simulink library "bcm"  (R2021b)
settings: Solver=VariableStepAuto  StartTime=0.0  StopTime=10.0  RelTol=1e-3
undefined symbols (not defined in the file or in its folder): ENUM_ANTITHEFT_ALARM, ENUM_ANTITHEFT_ARM, ENUM_ANTITHEFT_DISARM, ENUM_ANTITHEFT_WAIT, ENUM_GEARPOSNTOCAN_P, ENUM_PDKEYRAWLULOCK_INUNLOCK, ENUM_PDKEYRAWPS_INPS, ENUM_POWERSTA_ON, ENUM_POWERSTA_READY, ENUM_POWERSTA_STANDBY, FALSE, KBCM_ALMBrightnessDark_enum, KBCM_AmbBlue_enum, KBCM_AmbBreathT_ms, KBCM_AmbGreen_enum, KBCM_AmbRed_enum, KBCM_Antitheft_enum_ovrdflg, KBCM_Antitheft_enum_ovrdval, KBCM_APMDoorCtrlSta_flg_ovrdflg, KBCM_APMDoorCtrlSta_flg_ovrdval, KBCM_DelayTSW_flg, KBCM_DiagFLTC_mA, KBCM_DiagFMHT_s, KBCM_DiagFRTC_mA, KBCM_DiagRLTC_mA, KBCM_DiagRRTC_mA, KBCM_DrAPMRetryTimes_cnt, KBCM_DrOpenWdwOT_s, KBCM_DrOpenWdwReady_s, KBCM_ESSOffT_ms, KBCM_ESSOnT_ms, KBCM_IVIRstHoldT_ms, KBCM_IVIRstTriggerT_ms, KBCM_ONDelayT_ms, KBCM_ReDetectT_K, KBCM_RmLampKeep_min, KBCM_RmLpKeyInT_s, KBCM_RmLpKeyMissT_s, KBCM_SlpDebounceTime_s, KBCM_SPTGDetectT_sec, KBCM_SPTGLeave_flg, KBCM_SPTGLeftBound_cm, KBCM_SPTGLeftBoundOut_cm, KBCM_SPTGLowerBound_cm, KBCM_SPTGLowerBoundOut_cm, KBCM_SPTGRightBound_cm, KBCM_SPTGRightBoundOut_cm, KBCM_SPTGTOut_K, KBCM_SPTGUpperBound_cm, KBCM_SPTGUpperBoundOut_cm, KBCM_SPTGWaitDKC_sec, KBCM_TrunSWKeepTime3_s, KBCM_TrunSWKeepTime5_s, KBCM_TrunSWKeepTime7_s, KBCM_USSDis_cm, KBCM_USSFilterT_K, KBCM_WaitAPMPwr_K, KBCM_WdwManualDetT_s, MIN2SEC, TRUE ... (+1)
libraries: simulink x151, hcu_lib x5
(part 5 of 8)

== system bcm/BCM/BCM/PTG/KeyDetected ==
  VBCM_PASDRMR_cm : Inport
  VBCM_PASDRML_cm : Inport  Port=2
  AND{,1,3..4} (4 alike) : Logic  AllPortsSameDT=off  OutDataTypeStr=boolean
  AND2 : Logic  Inputs=3  AllPortsSameDT=off  OutDataTypeStr=boolean
  AND5 : Logic  Inputs=3  AllPortsSameDT=off  OutDataTypeStr=boolean
  Add : Sum
  Add1 : Sum  Inputs=-++
  Add2 : Sum  Inputs=--
  CheckSignalAvailable : Subsystem
  Compare To Constant2 : simulink/Logic and Bit Operations/Compare To Constant  relop=<=  const=KBCM_SPTGUpperBound_cm  OutDataTypeStr=boolean
  Compare To Constant3 : simulink/Logic and Bit Operations/Compare To Constant  relop=>=  const=KBCM_SPTGLowerBound_cm  OutDataTypeStr=boolean
  Constant : Constant  Value=KBCM_SPTGRightBound_cm
  Constant1 : Constant  Value=KBCM_USSFilterT_K
  Constant10 : Constant  Value=KBCM_USSDis_cm
  Constant11 : Constant  Value=KBCM_SPTGUpperBoundOut_cm
  Constant12 : Constant  Value=KBCM_SPTGLowerBoundOut_cm
  Constant13 : Constant  Value=KBCM_SPTGRightBoundOut_cm
  Constant14 : Constant  Value=KBCM_USSFilterT_K
  Constant15 : Constant  Value=-1  OutDataTypeStr=single
  Constant16 : Constant  Value=0  OutDataTypeStr=single
  Constant17 : Constant  Value=KBCM_SPTGUpperBound_cm
  Constant18 : Constant  Value=KBCM_SPTGLowerBound_cm
  Constant2 : Constant  Value=KBCM_SPTGLeftBound_cm
  Constant3 : Constant  Value=-1  OutDataTypeStr=single
  Constant4 : Constant  Value=KBCM_USSDis_cm
  Constant5 : Constant  Value=0  OutDataTypeStr=single
  Constant6 : Constant  Value=KBCM_SPTGLeftBoundOut_cm
  Constant7 : Constant  Value=KBCM_USSDis_cm
  Constant8 : Constant  Value=KBCM_SPTGLeftBound_cm
  Constant9 : Constant  Value=KBCM_SPTGLeftBound_cm
  Data Type Conversion : DataTypeConversion  OutDataTypeStr=single
  Data Type Conversion1 : DataTypeConversion  OutDataTypeStr=single
  Data Type Conversion2 : DataTypeConversion  OutDataTypeStr=boolean
  Data Type Conversion3 : DataTypeConversion  OutDataTypeStr=boolean
  Detect Decrease : simulink/Logic and Bit Operations/Detect Decrease  vinit=0.0  OutDataTypeStr=boolean
  Detect Decrease1 : simulink/Logic and Bit Operations/Detect Decrease  vinit=0.0  OutDataTypeStr=boolean
  Equal : RelationalOperator  OutDataTypeStr=boolean  RndMeth=Simplest
  Gain : Gain  Gain=-1
  GreaterThan : RelationalOperator  Operator=<=  OutDataTypeStr=boolean  RndMeth=Simplest
  GreaterThan1 : RelationalOperator  Operator=<=  OutDataTypeStr=boolean  RndMeth=Simplest
  GreaterThan2 : RelationalOperator  OutDataTypeStr=boolean  RndMeth=Simplest
  Less Than : RelationalOperator  Operator=<=  OutDataTypeStr=boolean  RndMeth=Simplest
  Less Than1 : RelationalOperator  OutDataTypeStr=boolean  RndMeth=Simplest
  Product : Product
  Sum1 : Sum
  Sum2 : Sum  Inputs=|++
  Sum3 : Sum  Inputs=|+-
  Sum4 : Sum
  Switch{1..6} (6 alike) : Switch  Criteria=u2 > Threshold
  Target_h : Subsystem
  Unit Delay{1..6} (6 alike) : UnitDelay  SampleTime=-1  HasFrameUpgradeWarning=on
  cosRML : Subsystem
  KeyDetected : Outport
  KeyDetectedOut : Outport  Port=2
  wires:
  Constant4/1 -> CheckSignalAvailable/3(KBCM_USSDis_cm_IN)
  CheckSignalAvailable/1(VBCM_PASDRML_cm) -> cosRML/1(VBCM_PASDRML_cm), Target_h/1(VBCM_PASDRML_cm), Product/2
  CheckSignalAvailable/2(VBCM_PASDRMR_cm) -> Target_h/2(VBCM_PASDRMR_cm), cosRML/2(VBCM_PASDRMR_cm)
  CheckSignalAvailable/3(KBCM_USSDis_cm) -> Target_h/3(KBCM_USSDis_cm), cosRML/3(KBCM_USSDis_cm)
  Target_h/1(Target_h) -> Less Than1/1, Less Than/1, Compare To Constant3/1, Compare To Constant2/1
  Compare To Constant2/1 -> AND1/1
  Compare To Constant3/1 -> AND1/2
  AND1/1 -> AND2/2
  AND/1 -> AND2/1
  cosRML/1(cosRML) -> Product/1
  CheckSignalAvailable/4(CheckResult) -> [CheckResult]
  [CheckResult] -> AND2/3
  Detect Decrease/1 -> Switch2/2
  Switch2/1 -> Data Type Conversion/1
  Constant1/1 -> Switch2/1
  Sum1/1 -> Switch2/3
  Unit Delay2/1 -> Switch3/2, Sum1/2, Switch4/2
  Constant3/1 -> Switch3/1
  Constant5/1 -> Switch3/3
  Switch3/1 -> Sum1/1
  Switch4/1 -> Data Type Conversion2/1, KeyDetected/1
  Unit Delay4/1 -> Switch4/1
  VBCM_PASDRML_cm/1 -> CheckSignalAvailable/1(VBCM_PASDRML_cm_IN)
  VBCM_PASDRMR_cm/1 -> CheckSignalAvailable/2(VBCM_PASDRMR_cm_IN)
  AND2/1 -> Unit Delay6/1, Detect Decrease/1
  GreaterThan1/1 -> AND4/1
  Add1/1 -> GreaterThan1/2
  [Target_x] -> GreaterThan2/1, GreaterThan1/1
  Product/1 -> [Target_x]
  [Target_x] -> GreaterThan/1, Equal/1
  Constant17/1 -> Sum2/1
  Constant11/1 -> Sum2/2
  Constant12/1 -> Sum3/2
  Constant18/1 -> Sum3/1
  [CheckResult] -> AND5/3
  AND3/1 -> AND5/1
  AND4/1 -> AND5/2
  AND5/1 -> Unit Delay1/1, Detect Decrease1/1
  Unit Delay5/1 -> Switch6/1
  Switch6/1 -> KeyDetectedOut/1, Data Type Conversion3/1
  Switch5/1 -> Sum4/1
  Constant16/1 -> Switch5/3
  Constant15/1 -> Switch5/1
  Unit Delay3/1 -> Switch6/2, Sum4/2, Switch5/2
  Sum4/1 -> Switch1/3
  Constant14/1 -> Switch1/1
  Switch1/1 -> Data Type Conversion1/1
  Detect Decrease1/1 -> Switch1/2
  Sum2/1 -> Less Than/2
  Less Than/1 -> AND3/1
  Sum3/1 -> Less Than1/2
  Less Than1/1 -> AND3/2
  Constant10/1 -> Add1/2
  Constant9/1 -> Add1/1
  Constant13/1 -> Add1/3
  Constant7/1 -> Add/2
  Equal/1 -> AND/1
  GreaterThan/1 -> AND/2
  Constant/1 -> Add/1
  Add/1 -> GreaterThan/2
  GreaterThan2/1 -> AND4/2
  Constant2/1 -> Add2/1
  Constant6/1 -> Add2/2
  Add2/1 -> GreaterThan2/2
  Unit Delay1/1 -> Switch6/3
  Unit Delay6/1 -> Switch4/3
  Constant8/1 -> Gain/1
  Gain/1 -> Equal/2
  Data Type Conversion/1 -> Unit Delay2/1
  Data Type Conversion1/1 -> Unit Delay3/1
  Data Type Conversion2/1 -> Unit Delay4/1
  Data Type Conversion3/1 -> Unit Delay5/1

== system bcm/BCM/BCM/PTG/Subsystem1 ==
  VAPM_PASDRMR_cm : Inport
  Add4 : Sum
  Compare To Constant1 : simulink/Logic and Bit Operations/Compare To Constant  relop=~=  const=0  OutDataTypeStr=boolean
  Compare To Constant6 : simulink/Logic and Bit Operations/Compare To Constant  relop===  const=0  OutDataTypeStr=boolean
  Compare To Constant8 : simulink/Logic and Bit Operations/Compare To Constant  relop===  const=255  OutDataTypeStr=boolean
  Constant1 : Constant  Value=0  OutDataTypeStr=uint8
  Constant12 : Constant  OutDataTypeStr=uint8
  Constant13 : Constant  Value=0  OutDataTypeStr=uint8
  Constant2 : Constant  OutDataTypeStr=uint8
  Constant3 : Constant  Value=KBCM_SPTGTOut_K
  Constant4 : Constant  Value=255  OutDataTypeStr=uint8
  Constant5 : Constant  Value=KBCM_SPTGTOut_K
  Detect Change : simulink/Logic and Bit Operations/Detect Change  vinit=0  OutDataTypeStr=boolean
  Equal : RelationalOperator  OutDataTypeStr=boolean  RndMeth=Simplest
  Equal1 : RelationalOperator  Operator===  OutDataTypeStr=boolean  RndMeth=Simplest
  Equal2 : RelationalOperator  Operator=~=  OutDataTypeStr=boolean  RndMeth=Simplest
  Logical Operator : Logic  Inputs=3  AllPortsSameDT=off  OutDataTypeStr=boolean
  Logical Operator2 : Logic  Operator=OR  AllPortsSameDT=off  OutDataTypeStr=boolean
  Switch{2..3,8..9} (4 alike) : Switch  Criteria=u2 > Threshold
  Unit Delay2 : UnitDelay  SampleTime=-1  HasFrameUpgradeWarning=on
  Unit Delay6 : UnitDelay  SampleTime=-1  HasFrameUpgradeWarning=on
  PASDRMR : Outport
  wires:
  Equal1/1 -> Logical Operator2/2
  Switch9/1 -> Add4/1
  Constant5/1 -> Equal1/1, Equal2/2
  Unit Delay6/1 -> Equal/1, Add4/2
  Compare To Constant8/1 -> Switch8/2
  Equal2/1 -> Logical Operator2/1
  Constant4/1 -> Switch3/3
  Switch2/1 -> Switch3/1, Unit Delay2/1
  Compare To Constant1/1 -> Logical Operator/2
  Logical Operator/1 -> Switch2/2
  Constant13/1 -> Switch9/1
  Add4/1 -> Switch8/1
  Unit Delay2/1 -> Switch2/3
  Constant12/1 -> Switch9/3
  Equal/1 -> Switch9/2
  Constant3/1 -> Equal/2
  Detect Change/1 -> Logical Operator/1
  Compare To Constant6/1 -> Logical Operator/3
  Constant1/1 -> Switch8/3
  Switch3/1 -> PASDRMR/1
  VAPM_PASDRMR_cm/1 -> Switch2/1, Detect Change/1, Compare To Constant1/1, Compare To Constant8/1
  Logical Operator2/1 -> Switch3/2
  Constant2/1 -> Equal1/2
  Switch8/1 -> Unit Delay6/1, Compare To Constant6/1, Equal2/1

== system bcm/BCM/BCM/PTG/Subsystem3 ==
  VAPM_PASDRML_cm : Inport
  Add4 : Sum
  Compare To Constant1 : simulink/Logic and Bit Operations/Compare To Constant  relop=~=  const=0  OutDataTypeStr=boolean
  Compare To Constant6 : simulink/Logic and Bit Operations/Compare To Constant  relop===  const=0  OutDataTypeStr=boolean
  Compare To Constant8 : simulink/Logic and Bit Operations/Compare To Constant  relop===  const=255  OutDataTypeStr=boolean
  Constant1 : Constant  Value=0  OutDataTypeStr=uint8
  Constant12 : Constant  OutDataTypeStr=uint8
  Constant13 : Constant  Value=0  OutDataTypeStr=uint8
  Constant2 : Constant  Value=0  OutDataTypeStr=uint8
  Constant3 : Constant  Value=KBCM_SPTGTOut_K
  Constant4 : Constant  Value=255  OutDataTypeStr=uint8
  Constant5 : Constant  Value=KBCM_SPTGTOut_K
  Detect Change : simulink/Logic and Bit Operations/Detect Change  vinit=0  OutDataTypeStr=boolean
  Equal : RelationalOperator  OutDataTypeStr=boolean  RndMeth=Simplest
  Equal1 : RelationalOperator  Operator===  OutDataTypeStr=boolean  RndMeth=Simplest
  Equal2 : RelationalOperator  Operator=~=  OutDataTypeStr=boolean  RndMeth=Simplest
  Logical Operator : Logic  Inputs=3  AllPortsSameDT=off  OutDataTypeStr=boolean
  Logical Operator2 : Logic  Operator=OR  AllPortsSameDT=off  OutDataTypeStr=boolean
  Switch{2..3,8..9} (4 alike) : Switch  Criteria=u2 > Threshold
  Unit Delay2 : UnitDelay  SampleTime=-1  HasFrameUpgradeWarning=on
  Unit Delay6 : UnitDelay  SampleTime=-1  HasFrameUpgradeWarning=on
  PASDRML : Outport
  wires:
  Constant2/1 -> Equal1/2
  Logical Operator2/1 -> Switch3/2
  VAPM_PASDRML_cm/1 -> Compare To Constant8/1, Compare To Constant1/1, Detect Change/1, Switch2/1
  Switch3/1 -> PASDRML/1
  Constant1/1 -> Switch8/3
  Compare To Constant6/1 -> Logical Operator/3
  Detect Change/1 -> Logical Operator/1
  Constant3/1 -> Equal/2
  Equal/1 -> Switch9/2
  Constant12/1 -> Switch9/3
  Unit Delay2/1 -> Switch2/3
  Add4/1 -> Switch8/1
  Constant13/1 -> Switch9/1
  Switch8/1 -> Equal2/1, Compare To Constant6/1, Unit Delay6/1
  Logical Operator/1 -> Switch2/2
  Compare To Constant1/1 -> Logical Operator/2
  Switch2/1 -> Unit Delay2/1, Switch3/1
  Constant4/1 -> Switch3/3
  Equal2/1 -> Logical Operator2/1
  Compare To Constant8/1 -> Switch8/2
  Unit Delay6/1 -> Add4/2, Equal/1
  Constant5/1 -> Equal2/2, Equal1/1
  Switch9/1 -> Add4/1
  Equal1/1 -> Logical Operator2/2

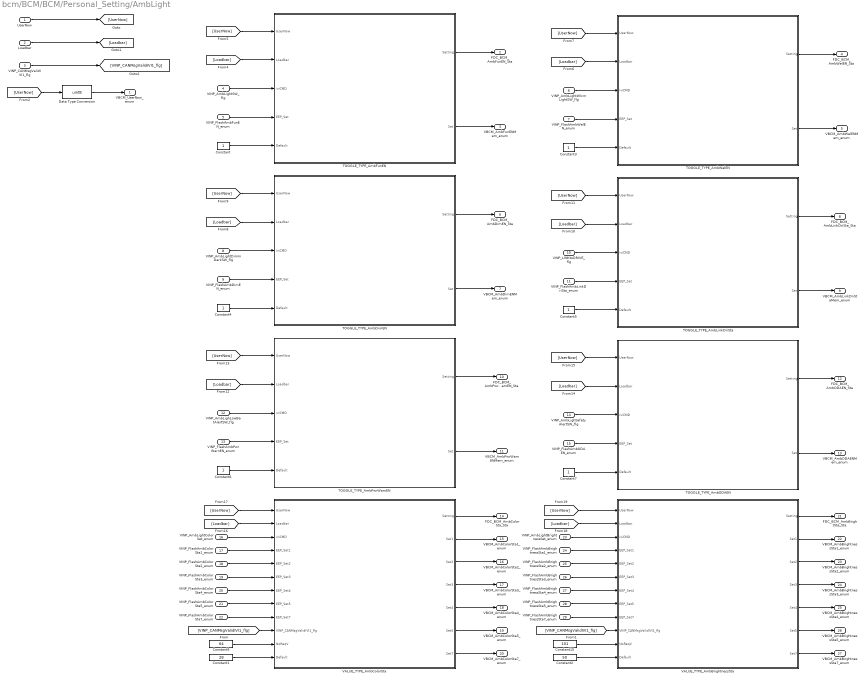
== system bcm/BCM/BCM/Personal_Setting/AmbLight ==
  UserNow : Inport
  Loadbar : Inport  Port=2
  VINP_CANMsgValidIVI1_flg : Inport  Port=3
  VINP_AmbLightSW_flg : Inport  Port=4
  VINP_FlashAmbFunEN_enum : Inport  Port=5
  VINP_AmbLightWlcmLightSW_flg : Inport  Port=6
  VINP_FlashAmbWelEN_enum : Inport  Port=7
  VINP_AmbLightDimInDarkSW_flg : Inport  Port=8
  VINP_FlashAmbDimEN_enum : Inport  Port=9
  VINP_LINKtoDRIVE_flg : Inport  Port=10
  VINP_FlashAmbLinkDriSta_enum : Inport  Port=11
  VINP_AmbLighLowBatAlertSW_flg : Inport  Port=12
  VINP_FlashAmbPwrWarnEN_enum : Inport  Port=13
  VINP_AmbLighSafetyAlertSW_flg : Inport  Port=14
  VINP_FlashAmbODAEN_enum : Inport  Port=15
  VINP_AmbLightColorSet_enum : Inport  Port=16
  VINP_FlashAmbColorSta1_enum : Inport  Port=17
  VINP_FlashAmbColorSta2_enum : Inport  Port=18
  VINP_FlashAmbColorSta3_enum : Inport  Port=19
  VINP_FlashAmbColorSta4_enum : Inport  Port=20
  VINP_FlashAmbColorSta5_enum : Inport  Port=21
  VINP_FlashAmbColorSta7_enum : Inport  Port=22
  VINP_AmbLightBrightnessSet_enum : Inport  Port=23
  VINP_FlashAmbBrightnessSta1_enum : Inport  Port=24
  VINP_FlashAmbBrightnessSta2_enum : Inport  Port=25
  VINP_FlashAmbBrightnessSta3_enum : Inport  Port=26
  VINP_FlashAmbBrightnessSta4_enum : Inport  Port=27
  VINP_FlashAmbBrightnessSta5_enum : Inport  Port=28
  VINP_FlashAmbBrightnessSta7_enum : Inport  Port=29
  Constant{,3..7} (6 alike) : Constant  OutDataTypeStr=boolean
  Constant1 : Constant  Value=28  OutDataTypeStr=uint8
  Constant10 : Constant  Value=101  OutDataTypeStr=uint8
  Constant2 : Constant  Value=50  OutDataTypeStr=uint8
  Constant9 : Constant  Value=64  OutDataTypeStr=uint8
  Data Type Conversion : DataTypeConversion  OutDataTypeStr=uint8
  TOGGLE_TYPE_AmbDimEN : Subsystem
  TOGGLE_TYPE_AmbFunEN : Subsystem
  TOGGLE_TYPE_AmbLinkDriSta : Subsystem
  TOGGLE_TYPE_AmbODAEN : Subsystem
  TOGGLE_TYPE_AmbPwrWarnEN : Subsystem
  TOGGLE_TYPE_AmbWelEN : Subsystem
  VALUE_TYPE_AmbBrightnessSta : Subsystem
  VALUE_TYPE_AmbColorSta : Subsystem
  VBCM_UserNow_enum : Outport
  FDC_BCM_AmbFunEN_Sta : Outport  Port=2
  VBCM_AmbFunENMem_enum : Outport  Port=3
  FDC_BCM_AmbWelEN_Sta : Outport  Port=4
  VBCM_AmbWelENMem_enum : Outport  Port=5
  FDC_BCM_AmbDimEN_Sta : Outport  Port=6
  VBCM_AmbDimENMem_enum : Outport  Port=7
  FDC_BCM_AmbLinkDriSta_Sta : Outport  Port=8
  VBCM_AmbLinkDriStaMem_enum : Outport  Port=9
  FDC_BCM_AmbPwrWarnEN_Sta : Outport  Port=10
  VBCM_AmbPwrWarnENMem_enum : Outport  Port=11
  FDC_BCM_AmbODAEN_Sta : Outport  Port=12
  VBCM_AmbODAENMem_enum : Outport  Port=13
  FDC_BCM_AmbColorSta_Sta : Outport  Port=14
  VBCM_AmbColorSta1_enum : Outport  Port=15
  VBCM_AmbColorSta2_enum : Outport  Port=16
  VBCM_AmbColorSta3_enum : Outport  Port=17
  VBCM_AmbColorSta4_enum : Outport  Port=18
  VBCM_AmbColorSta5_enum : Outport  Port=19
  VBCM_AmbColorSta7_enum : Outport  Port=20
  FDC_BCM_AmbBrightSta_Sta : Outport  Port=21  OutDataTypeStr=uint8
  VBCM_AmbBrightnessSta1_enum : Outport  Port=22  OutDataTypeStr=uint8
  VBCM_AmbBrightnessSta2_enum : Outport  Port=23
  VBCM_AmbBrightnessSta3_enum : Outport  Port=24
  VBCM_AmbBrightnessSta4_enum : Outport  Port=25
  VBCM_AmbBrightnessSta5_enum : Outport  Port=26
  VBCM_AmbBrightnessSta7_enum : Outport  Port=27
  wires:
  VALUE_TYPE_AmbBrightnessSta/3(Set2) -> VBCM_AmbBrightnessSta2_enum/1
  VALUE_TYPE_AmbBrightnessSta/2(Set1) -> VBCM_AmbBrightnessSta1_enum/1
  [UserNow] -> VALUE_TYPE_AmbBrightnessSta/1(UserNow)
  VALUE_TYPE_AmbBrightnessSta/1(Setting) -> FDC_BCM_AmbBrightSta_Sta/1
  TOGGLE_TYPE_AmbFunEN/1(Setting) -> FDC_BCM_AmbFunEN_Sta/1
  [Loadbar] -> VALUE_TYPE_AmbColorSta/2(Loadbar)
  VALUE_TYPE_AmbBrightnessSta/6(Set5) -> VBCM_AmbBrightnessSta5_enum/1
  TOGGLE_TYPE_AmbFunEN/2(Set) -> VBCM_AmbFunENMem_enum/1
  VALUE_TYPE_AmbBrightnessSta/7(Set7) -> VBCM_AmbBrightnessSta7_enum/1
  VALUE_TYPE_AmbBrightnessSta/4(Set3) -> VBCM_AmbBrightnessSta3_enum/1
  [UserNow] -> VALUE_TYPE_AmbColorSta/1(UserNow)
  VALUE_TYPE_AmbBrightnessSta/5(Set4) -> VBCM_AmbBrightnessSta4_enum/1
  [Loadbar] -> VALUE_TYPE_AmbBrightnessSta/2(Loadbar)
  UserNow/1 -> [UserNow]
  Loadbar/1 -> [Loadbar]
  VALUE_TYPE_AmbColorSta/1(Setting) -> FDC_BCM_AmbColorSta_Sta/1
  VALUE_TYPE_AmbColorSta/2(Set1) -> VBCM_AmbColorSta1_enum/1
  VALUE_TYPE_AmbColorSta/3(Set2) -> VBCM_AmbColorSta2_enum/1
  VALUE_TYPE_AmbColorSta/4(Set3) -> VBCM_AmbColorSta3_enum/1
  VALUE_TYPE_AmbColorSta/5(Set4) -> VBCM_AmbColorSta4_enum/1
  VALUE_TYPE_AmbColorSta/6(Set5) -> VBCM_AmbColorSta5_enum/1
  VALUE_TYPE_AmbColorSta/7(Set7) -> VBCM_AmbColorSta7_enum/1
  [UserNow] -> TOGGLE_TYPE_AmbFunEN/1(UserNow)
  [Loadbar] -> TOGGLE_TYPE_AmbFunEN/2(Loadbar)
  VINP_AmbLightSW_flg/1 -> TOGGLE_TYPE_AmbFunEN/3(iviCMD)
  VINP_FlashAmbFunEN_enum/1 -> TOGGLE_TYPE_AmbFunEN/4(EEP_Set)
  Constant/1 -> TOGGLE_TYPE_AmbFunEN/5(Default)
  Constant9/1 -> VALUE_TYPE_AmbColorSta/11(NoReqV)
  Constant1/1 -> VALUE_TYPE_AmbColorSta/12(Default)
  VINP_FlashAmbColorSta7_enum/1 -> VALUE_TYPE_AmbColorSta/9(EEP_Set7)
  VINP_FlashAmbColorSta5_enum/1 -> VALUE_TYPE_AmbColorSta/8(EEP_Set5)
  VINP_FlashAmbColorSta4_enum/1 -> VALUE_TYPE_AmbColorSta/7(EEP_Set4)
  VINP_FlashAmbColorSta3_enum/1 -> VALUE_TYPE_AmbColorSta/6(EEP_Set3)
  VINP_FlashAmbColorSta2_enum/1 -> VALUE_TYPE_AmbColorSta/5(EEP_Set2)
  VINP_FlashAmbColorSta1_enum/1 -> VALUE_TYPE_AmbColorSta/4(EEP_Set1)
  VINP_AmbLightColorSet_enum/1 -> VALUE_TYPE_AmbColorSta/3(iviCMD)
  Constant10/1 -> VALUE_TYPE_AmbBrightnessSta/11(NoReqV)
  Constant2/1 -> VALUE_TYPE_AmbBrightnessSta/12(Default)
  VINP_FlashAmbBrightnessSta7_enum/1 -> VALUE_TYPE_AmbBrightnessSta/9(EEP_Set7)
  VINP_FlashAmbBrightnessSta5_enum/1 -> VALUE_TYPE_AmbBrightnessSta/8(EEP_Set5)
  VINP_FlashAmbBrightnessSta4_enum/1 -> VALUE_TYPE_AmbBrightnessSta/7(EEP_Set4)
  VINP_FlashAmbBrightnessSta3_enum/1 -> VALUE_TYPE_AmbBrightnessSta/6(EEP_Set3)
  VINP_FlashAmbBrightnessSta2_enum/1 -> VALUE_TYPE_AmbBrightnessSta/5(EEP_Set2)
  VINP_FlashAmbBrightnessSta1_enum/1 -> VALUE_TYPE_AmbBrightnessSta/4(EEP_Set1)
  VINP_AmbLightBrightnessSet_enum/1 -> VALUE_TYPE_AmbBrightnessSta/3(iviCMD)
  [UserNow] -> TOGGLE_TYPE_AmbWelEN/1(UserNow)
  [Loadbar] -> TOGGLE_TYPE_AmbWelEN/2(Loadbar)
  Constant3/1 -> TOGGLE_TYPE_AmbWelEN/5(Default)
  VINP_AmbLightWlcmLightSW_flg/1 -> TOGGLE_TYPE_AmbWelEN/3(iviCMD)
  VINP_FlashAmbWelEN_enum/1 -> TOGGLE_TYPE_AmbWelEN/4(EEP_Set)
  TOGGLE_TYPE_AmbWelEN/1(Setting) -> FDC_BCM_AmbWelEN_Sta/1
  TOGGLE_TYPE_AmbWelEN/2(Set) -> VBCM_AmbWelENMem_enum/1
  [UserNow] -> TOGGLE_TYPE_AmbDimEN/1(UserNow)
  Constant4/1 -> TOGGLE_TYPE_AmbDimEN/5(Default)
  [Loadbar] -> TOGGLE_TYPE_AmbDimEN/2(Loadbar)
  VINP_AmbLightDimInDarkSW_flg/1 -> TOGGLE_TYPE_AmbDimEN/3(iviCMD)
  VINP_FlashAmbDimEN_enum/1 -> TOGGLE_TYPE_AmbDimEN/4(EEP_Set)
  TOGGLE_TYPE_AmbDimEN/1(Setting) -> FDC_BCM_AmbDimEN_Sta/1
  TOGGLE_TYPE_AmbDimEN/2(Set) -> VBCM_AmbDimENMem_enum/1
  [UserNow] -> TOGGLE_TYPE_AmbLinkDriSta/1(UserNow)
  Constant5/1 -> TOGGLE_TYPE_AmbLinkDriSta/5(Default)
  [Loadbar] -> TOGGLE_TYPE_AmbLinkDriSta/2(Loadbar)
  VINP_LINKtoDRIVE_flg/1 -> TOGGLE_TYPE_AmbLinkDriSta/3(iviCMD)
  VINP_FlashAmbLinkDriSta_enum/1 -> TOGGLE_TYPE_AmbLinkDriSta/4(EEP_Set)
  TOGGLE_TYPE_AmbLinkDriSta/1(Setting) -> FDC_BCM_AmbLinkDriSta_Sta/1
  TOGGLE_TYPE_AmbLinkDriSta/2(Set) -> VBCM_AmbLinkDriStaMem_enum/1
  Constant6/1 -> TOGGLE_TYPE_AmbPwrWarnEN/5(Default)
  [UserNow] -> TOGGLE_TYPE_AmbPwrWarnEN/1(UserNow)
  [Loadbar] -> TOGGLE_TYPE_AmbPwrWarnEN/2(Loadbar)
  VINP_AmbLighLowBatAlertSW_flg/1 -> TOGGLE_TYPE_AmbPwrWarnEN/3(iviCMD)
  VINP_FlashAmbPwrWarnEN_enum/1 -> TOGGLE_TYPE_AmbPwrWarnEN/4(EEP_Set)
  TOGGLE_TYPE_AmbPwrWarnEN/1(Setting) -> FDC_BCM_AmbPwrWarnEN_Sta/1
  TOGGLE_TYPE_AmbPwrWarnEN/2(Set) -> VBCM_AmbPwrWarnENMem_enum/1
  [UserNow] -> TOGGLE_TYPE_AmbODAEN/1(UserNow)
  [Loadbar] -> TOGGLE_TYPE_AmbODAEN/2(Loadbar)
  Constant7/1 -> TOGGLE_TYPE_AmbODAEN/5(Default)
  VINP_AmbLighSafetyAlertSW_flg/1 -> TOGGLE_TYPE_AmbODAEN/3(iviCMD)
  VINP_FlashAmbODAEN_enum/1 -> TOGGLE_TYPE_AmbODAEN/4(EEP_Set)
  TOGGLE_TYPE_AmbODAEN/1(Setting) -> FDC_BCM_AmbODAEN_Sta/1
  TOGGLE_TYPE_AmbODAEN/2(Set) -> VBCM_AmbODAENMem_enum/1
  VINP_CANMsgValidIVI1_flg/1 -> [VINP_CANMsgValidIVI1_flg]
  [VINP_CANMsgValidIVI1_flg] -> VALUE_TYPE_AmbColorSta/10(VINP_CANMsgValidIVI1_flg)
  [VINP_CANMsgValidIVI1_flg] -> VALUE_TYPE_AmbBrightnessSta/10(VINP_CANMsgValidIVI1_flg)
  [UserNow] -> Data Type Conversion/1
  Data Type Conversion/1 -> VBCM_UserNow_enum/1

== system bcm/BCM/BCM/Personal_Setting/System_Loadbar ==
  Add : Sum
  Compare To Constant : simulink/Logic and Bit Operations/Compare To Constant  relop=>  const=2  OutDataTypeStr=boolean
  Constant6 : Constant  Value=0  OutDataTypeStr=uint8
  Constant7 : Constant  OutDataTypeStr=uint8
  Switch7 : Switch  Criteria=u2 > Threshold
  Unit Delay : UnitDelay  SampleTime=-1  HasFrameUpgradeWarning=on
  Unit Delay6 : UnitDelay  SampleTime=-1  HasFrameUpgradeWarning=on
  Loadbar : Outport
  wires:
  Constant7/1 -> Switch7/3
  Unit Delay6/1 -> Add/1
  Switch7/1 -> Add/2
  Unit Delay/1 -> Switch7/2
  Compare To Constant/1 -> Unit Delay/1, Loadbar/1
  Add/1 -> Unit Delay6/1, Compare To Constant/1
  Constant6/1 -> Switch7/1

== system bcm/BCM/BCM/PTG/KeyDetected/CheckSignalAvailable ==
  VBCM_PASDRML_cm_IN : Inport
  VBCM_PASDRMR_cm_IN : Inport  Port=2
  KBCM_USSDis_cm_IN : Inport  Port=3
  AND : Logic  Inputs=3  AllPortsSameDT=off  OutDataTypeStr=boolean
  Constant : Constant  OutDataTypeStr=single
  Constant1 : Constant  OutDataTypeStr=single
  Constant2 : Constant  OutDataTypeStr=single
  Constant3 : Constant  Value=KBCM_SPTGLowerBound_cm
  Constant4 : Constant  Value=KBCM_SPTGLowerBoundOut_cm
  Constant5 : Constant  Value=KBCM_SPTGLowerBound_cm
  Constant6 : Constant  Value=KBCM_SPTGLowerBoundOut_cm
  Demux : Demux  Outputs=3
  Equal : RelationalOperator  OutDataTypeStr=boolean  RndMeth=Simplest
  Equal1 : RelationalOperator  OutDataTypeStr=boolean  RndMeth=Simplest
  GreaterThan : RelationalOperator  OutDataTypeStr=boolean  RndMeth=Simplest
  Max : MinMax  Function=max  Inputs=3
  Mux : Mux  Inputs=3
  Mux1 : Mux  Inputs=3
  Sum : Sum  Inputs=+-
  Sum1 : Sum  Inputs=+++
  Sum2 : Sum  Inputs=|+-
  Sum3 : Sum  Inputs=|+-
  Switch : Switch  Criteria=u2 > Threshold
  VBCM_PASDRML_cm : Outport
  VBCM_PASDRMR_cm : Outport  Port=2
  KBCM_USSDis_cm : Outport  Port=3
  CheckResult : Outport  Port=4
  wires:
  GreaterThan/1 -> AND/1
  VBCM_PASDRML_cm_IN/1 -> [VBCM_PASDRML_cm_IN]
  VBCM_PASDRMR_cm_IN/1 -> [VBCM_PASDRMR_cm_IN]
  KBCM_USSDis_cm_IN/1 -> [KBCM_USSDis_cm_IN]
  AND/1 -> Switch/2, CheckResult/1
  Mux/1 -> Switch/1
  [VBCM_PASDRML_cm_IN] -> Mux/1
  [VBCM_PASDRMR_cm_IN] -> Mux/2
  [KBCM_USSDis_cm_IN] -> Mux/3
  Mux1/1 -> Switch/3
  Constant/1 -> Mux1/1
  Constant1/1 -> Mux1/2
  Switch/1 -> Demux/1
  Demux/1 -> VBCM_PASDRML_cm/1
  Demux/2 -> VBCM_PASDRMR_cm/1
  Demux/3 -> KBCM_USSDis_cm/1
  Equal/1 -> AND/2
  [VBCM_PASDRML_cm_IN] -> Max/1, Sum1/1
  [VBCM_PASDRMR_cm_IN] -> Max/2, Sum1/2
  [KBCM_USSDis_cm_IN] -> Max/3, Sum1/3
  Sum1/1 -> Sum/1
  Max/1 -> Sum/2, GreaterThan/2
  Sum/1 -> GreaterThan/1
  Constant2/1 -> Mux1/3
  Equal1/1 -> AND/3
  [VBCM_PASDRMR_cm_IN] -> Equal/1
  Constant3/1 -> Sum2/1
  Constant4/1 -> Sum2/2
  Sum2/1 -> Equal/2
  Sum3/1 -> Equal1/2
  Constant6/1 -> Sum3/2
  Constant5/1 -> Sum3/1
  [VBCM_PASDRML_cm_IN] -> Equal1/1

== system bcm/BCM/BCM/PTG/KeyDetected/Target_h ==
  VBCM_PASDRML_cm : Inport
  VBCM_PASDRMR_cm : Inport  Port=2
  KBCM_USSDis_cm : Inport  Port=3
  Data Type Conversion : DataTypeConversion
  Divide : Product  Inputs=*/
  Gain : Gain  Gain=2
  Gain1 : Gain  Gain=0.5
  Product : Product  Inputs=4
  Sqrt1 : Sqrt  SaturateOnIntegerOverflow=on
  Sum : Sum  Inputs=+-
  Sum1 : Sum  Inputs=+++
  Sum2 : Sum  Inputs=+-
  Sum3 : Sum  Inputs=+-
  Terminator : Terminator
  Target_h : Outport
  wires:
  Divide/1 -> Data Type Conversion/1, Target_h/1
  VBCM_PASDRML_cm/1 -> Sum/2, Sum1/1
  VBCM_PASDRMR_cm/1 -> Sum2/2, Sum1/2
  KBCM_USSDis_cm/1 -> Divide/2, Sum3/2, Sum1/3
  Sum1/1 -> Gain1/1
  Sum/1 -> Product/2
  Sum2/1 -> Product/3
  Sum3/1 -> Product/4
  Product/1 -> Sqrt1/1
  Sqrt1/1 -> Gain/1
  Gain/1 -> Divide/1
  Gain1/1 -> Sum3/1, Sum2/1, Sum/1, Product/1
  Data Type Conversion/1 -> Terminator/1  "VBCM_Targeth_cm"

== system bcm/BCM/BCM/PTG/KeyDetected/cosRML ==
  VBCM_PASDRML_cm : Inport
  VBCM_PASDRMR_cm : Inport  Port=2
  KBCM_USSDis_cm : Inport  Port=3
  Divide : Product  Inputs=*/
  Gain : Gain  Gain=2
  Product : Product
  Square : Math  Operator=square  SaturateOnIntegerOverflow=on
  Square1 : Math  Operator=square  SaturateOnIntegerOverflow=on
  Square2 : Math  Operator=square  SaturateOnIntegerOverflow=on
  Sum : Sum  Inputs=+-+
  cosRML : Outport
  wires:
  VBCM_PASDRML_cm/1 -> Product/1, Square/1
  VBCM_PASDRMR_cm/1 -> Square1/1
  KBCM_USSDis_cm/1 -> Product/2, Square2/1
  Square/1 -> Sum/1
  Square1/1 -> Sum/2
  Square2/1 -> Sum/3
  Product/1 -> Gain/1
  Sum/1 -> Divide/1
  Divide/1 -> cosRML/1
  Gain/1 -> Divide/2

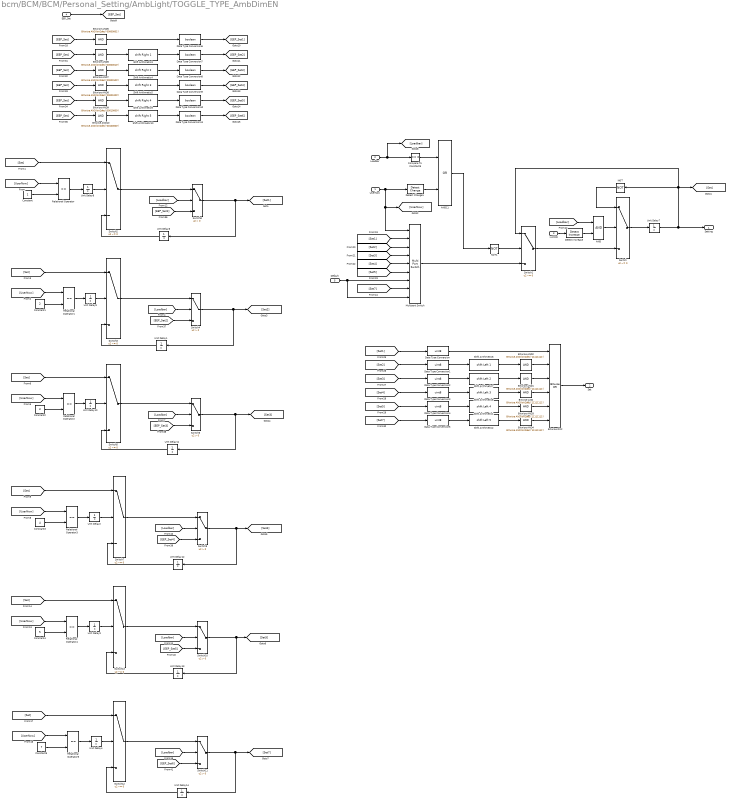
== system bcm/BCM/BCM/Personal_Setting/AmbLight/TOGGLE_TYPE_AmbDimEN ==
  UserNow : Inport
  Loadbar : Inport  Port=2
  iviCMD : Inport  Port=3
  EEP_Set : Inport  Port=4
  Default : Inport  Port=5
  AND : Logic  AllPortsSameDT=off  OutDataTypeStr=boolean
  AND11 : Logic  Operator=OR  AllPortsSameDT=off  OutDataTypeStr=boolean
  Bitwise AND{,1..4} (5 alike) : simulink/Logic and Bit Operations/Bitwise Operator  logicop=AND  UseBitMask=on  BitMask=bin2dec('11111111')  BitMaskRealWorld=Stored Integer
  Bitwise AND10 : simulink/Logic and Bit Operations/Bitwise Operator  logicop=AND  UseBitMask=on  BitMask=bin2dec('00100000')  BitMaskRealWorld=Stored Integer
  Bitwise AND5 : simulink/Logic and Bit Operations/Bitwise Operator  logicop=AND  UseBitMask=on  BitMask=bin2dec('00000001')  BitMaskRealWorld=Stored Integer
  Bitwise AND6 : simulink/Logic and Bit Operations/Bitwise Operator  logicop=AND  UseBitMask=on  BitMask=bin2dec('00000010')  BitMaskRealWorld=Stored Integer
  Bitwise AND7 : simulink/Logic and Bit Operations/Bitwise Operator  logicop=AND  UseBitMask=on  BitMask=bin2dec('00000100')  BitMaskRealWorld=Stored Integer
  Bitwise AND8 : simulink/Logic and Bit Operations/Bitwise Operator  logicop=AND  UseBitMask=on  BitMask=bin2dec('00001000')  BitMaskRealWorld=Stored Integer
  Bitwise AND9 : simulink/Logic and Bit Operations/Bitwise Operator  logicop=AND  UseBitMask=on  BitMask=bin2dec('00010000')  BitMaskRealWorld=Stored Integer
  Bitwise OR2 : simulink/Logic and Bit Operations/Bitwise Operator  logicop=OR  UseBitMask=off  NumInputPorts=6  BitMask=bin2dec('00000000000000000000')  BitMaskRealWorld=Stored Integer
  Compare To Constant5 : simulink/Logic and Bit Operations/Compare To Constant  relop===  const=0  OutDataTypeStr=boolean
  Constant : Constant  OutDataTypeStr=uint8
  Constant1 : Constant  Value=2  OutDataTypeStr=uint8
  Constant2 : Constant  Value=3  OutDataTypeStr=uint8
  Constant3 : Constant  Value=4  OutDataTypeStr=uint8
  Constant4 : Constant  Value=5  OutDataTypeStr=uint8
  Constant5 : Constant  Value=7  OutDataTypeStr=uint8
  Data Type Conversion{,1..5} (6 alike) : DataTypeConversion  OutDataTypeStr=uint8
  Data Type Conversion{6..11} (6 alike) : DataTypeConversion  OutDataTypeStr=boolean
  Detect Change1 : simulink/Logic and Bit Operations/Detect Change  vinit=0  OutDataTypeStr=boolean
  Detect Increase : simulink/Logic and Bit Operations/Detect Increase  vinit=0.0  OutDataTypeStr=boolean
  Multiport Switch : MultiPortSwitch  Inputs=7  DataPortForDefault=Additional data port  DiagnosticForDefault=None
  NOT : Logic  Operator=NOT  IconShape=distinctive  AllPortsSameDT=off  OutDataTypeStr=boolean
  NOT1 : Logic  Operator=NOT  IconShape=distinctive  AllPortsSameDT=off  OutDataTypeStr=boolean
  Relational Operator{,1..5} (6 alike) : RelationalOperator  Operator===  OutDataTypeStr=boolean  RndMeth=Simplest
  Shift Arithmetic1 : ArithShift  BitShiftNumber=4  BitShiftDirection=Left
  Shift Arithmetic10 : ArithShift  BitShiftNumber=5  BitShiftDirection=Right
  Shift Arithmetic2 : ArithShift  BitShiftNumber=5  BitShiftDirection=Left
  Shift Arithmetic3 : ArithShift  BitShiftNumber=1  BitShiftDirection=Right
  Shift Arithmetic4 : ArithShift  BitShiftNumber=2  BitShiftDirection=Right
  Shift Arithmetic5 : ArithShift  BitShiftNumber=3  BitShiftDirection=Right
  Shift Arithmetic6 : ArithShift  BitShiftNumber=1  BitShiftDirection=Left
  Shift Arithmetic7 : ArithShift  BitShiftNumber=2  BitShiftDirection=Left
  Shift Arithmetic8 : ArithShift  BitShiftNumber=3  BitShiftDirection=Left
  Shift Arithmetic9 : ArithShift  BitShiftNumber=4  BitShiftDirection=Right
  Switch{,1..3,5,7,12..13} (8 alike) : Switch  Criteria=u2 ~= 0
  Switch{4,6,8..11} (6 alike) : Switch  Criteria=u2 > Threshold
  Unit Delay{1..4,6..14} (13 alike) : UnitDelay  SampleTime=-1  HasFrameUpgradeWarning=on
  Setting : Outport
  Set : Outport  Port=2
  wires:
  [Loadbar] -> AND/1
  Detect Increase/1 -> AND/2
  AND/1 -> Switch/2
  Unit Delay14/1 -> Switch12/3
  Unit Delay4/1 -> Switch12/2
  Unit Delay13/1 -> Switch13/3
  Unit Delay3/1 -> Switch13/2
  Unit Delay12/1 -> Switch7/3
  Unit Delay2/1 -> Switch7/2
  Unit Delay11/1 -> Switch5/3
  Unit Delay10/1 -> Switch5/2
  Unit Delay9/1 -> Switch3/2
  Unit Delay8/1 -> Switch2/2
  Unit Delay1/1 -> Switch3/3
  Unit Delay6/1 -> Switch2/3
  Relational Operator1/1 -> Unit Delay9/1
  Relational Operator/1 -> Unit Delay8/1
  [EEP_Set6] -> Switch11/3
  [EEP_Set5] -> Switch10/3
  [EEP_Set4] -> Switch9/3
  [EEP_Set3] -> Switch6/3
  [EEP_Set2] -> Switch4/3
  [EEP_Set1] -> Switch8/3
  Data Type Conversion11/1 -> [EEP_Set6]
  Data Type Conversion10/1 -> [EEP_Set5]
  Data Type Conversion9/1 -> [EEP_Set4]
  Data Type Conversion8/1 -> [EEP_Set3]
  Data Type Conversion7/1 -> [EEP_Set2]
  Data Type Conversion6/1 -> [EEP_Set1]
  [EEP_Set] -> Bitwise AND10/1
  [EEP_Set] -> Bitwise AND9/1
  [EEP_Set] -> Bitwise AND8/1
  [EEP_Set] -> Bitwise AND7/1
  [EEP_Set] -> Bitwise AND6/1
  [EEP_Set] -> Bitwise AND5/1
  EEP_Set/1 -> [EEP_Set]
  Shift Arithmetic5/1 -> Data Type Conversion9/1
  Shift Arithmetic9/1 -> Data Type Conversion10/1
  Bitwise AND7/1 -> Shift Arithmetic4/1
  Shift Arithmetic3/1 -> Data Type Conversion7/1
  Bitwise AND5/1 -> Data Type Conversion6/1
  Shift Arithmetic10/1 -> Data Type Conversion11/1
  Shift Arithmetic4/1 -> Data Type Conversion8/1
  Bitwise AND10/1 -> Shift Arithmetic10/1
  Bitwise AND9/1 -> Shift Arithmetic9/1
  Bitwise AND6/1 -> Shift Arithmetic3/1
  Bitwise AND8/1 -> Shift Arithmetic5/1
  Bitwise OR2/1 -> Set/1
  [Set3] -> Data Type Conversion2/1
  Bitwise AND4/1 -> Bitwise OR2/6
  Data Type Conversion1/1 -> Shift Arithmetic6/1
  Bitwise AND/1 -> Bitwise OR2/4
  [Set5] -> Data Type Conversion4/1
  [Set1] -> Data Type Conversion/1
  Data Type Conversion3/1 -> Shift Arithmetic8/1
  [Set2] -> Data Type Conversion1/1
  Data Type Conversion/1 -> Bitwise OR2/1
  [Set7] -> Data Type Conversion5/1
  Shift Arithmetic1/1 -> Bitwise AND3/1
  Shift Arithmetic7/1 -> Bitwise AND1/1
  Data Type Conversion4/1 -> Shift Arithmetic1/1
  Shift Arithmetic6/1 -> Bitwise AND2/1
  Bitwise AND2/1 -> Bitwise OR2/2
  Bitwise AND1/1 -> Bitwise OR2/3
  Bitwise AND3/1 -> Bitwise OR2/5
  Shift Arithmetic2/1 -> Bitwise AND4/1
  Shift Arithmetic8/1 -> Bitwise AND/1
  [Set4] -> Data Type Conversion3/1
  Data Type Conversion5/1 -> Shift Arithmetic2/1
  Data Type Conversion2/1 -> Shift Arithmetic7/1
  Relational Operator5/1 -> Unit Delay4/1
  Relational Operator4/1 -> Unit Delay3/1
  Relational Operator3/1 -> Unit Delay2/1
  Relational Operator2/1 -> Unit Delay10/1
  Unit Delay7/1 -> Switch1/1, [Set], NOT/1, Setting/1
  Switch11/1 -> Unit Delay14/1, [Set7]
  Switch12/1 -> Switch11/1
  Switch10/1 -> Unit Delay13/1, [Set5]
  Switch9/1 -> Unit Delay12/1, [Set4]
  Switch7/1 -> Switch9/1
  Switch5/1 -> Switch6/1
  Switch6/1 -> Unit Delay11/1, [Set3]
  Switch4/1 -> Unit Delay1/1, [Set2]
  Switch3/1 -> Switch4/1
  Switch2/1 -> Switch8/1
  Switch8/1 -> Unit Delay6/1, [Set1]
  Switch/1 -> Unit Delay7/1
  AND11/1 -> NOT1/1
  Compare To Constant5/1 -> AND11/1
  Constant4/1 -> Relational Operator4/2
  [Loadbar] -> Switch8/2
  [Set] -> Switch5/1
  [Loadbar] -> Switch6/2
  [Set] -> Switch7/1
  Constant1/1 -> Relational Operator1/2
  [UserNow] -> Relational Operator4/1
  [Set] -> Switch2/1
  Constant3/1 -> Relational Operator3/2
  [UserNow] -> Relational Operator3/1
  [UserNow] -> Relational Operator2/1
  [Loadbar] -> Switch9/2
  Constant/1 -> Relational Operator/2
  [Set] -> Switch3/1
  [Loadbar] -> Switch11/2
  Constant2/1 -> Relational Operator2/2
  [Loadbar] -> Switch10/2
  [UserNow] -> Relational Operator1/1
  [UserNow] -> Relational Operator/1
  Constant5/1 -> Relational Operator5/2
  [UserNow] -> Relational Operator5/1
  [Set] -> Switch12/1
  [Loadbar] -> Switch4/2
  [Set] -> Switch13/1
  iviCMD/1 -> Detect Increase/1
  NOT/1 -> Switch/1
  UserNow/1 -> Detect Change1/1, [UserNow], Multiport Switch/1
  Switch1/1 -> Switch/3
  Loadbar/1 -> Compare To Constant5/1, [Loadbar]
  Multiport Switch/1 -> Switch1/3
  Detect Change1/1 -> AND11/2
  Switch13/1 -> Switch10/1
  NOT1/1 -> Switch1/2
  [Set1] -> Multiport Switch/2
  [Set2] -> Multiport Switch/3
  [Set3] -> Multiport Switch/4
  [Set4] -> Multiport Switch/5
  [Set5] -> Multiport Switch/6
  [Set7] -> Multiport Switch/8
  Default/1 -> Multiport Switch/9, Multiport Switch/7

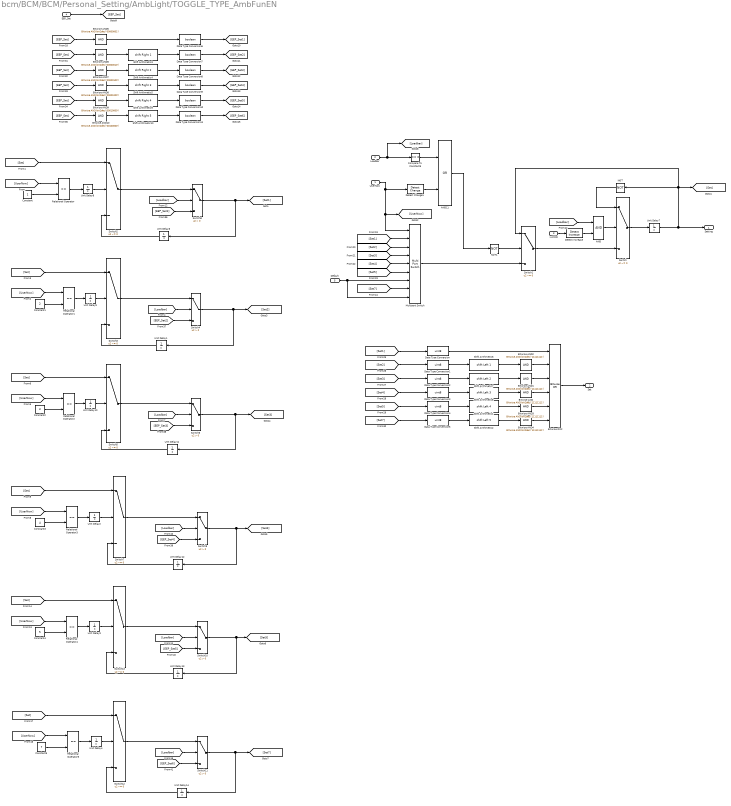
== system bcm/BCM/BCM/Personal_Setting/AmbLight/TOGGLE_TYPE_AmbFunEN ==
  UserNow : Inport
  Loadbar : Inport  Port=2
  iviCMD : Inport  Port=3
  EEP_Set : Inport  Port=4
  Default : Inport  Port=5
  AND : Logic  AllPortsSameDT=off  OutDataTypeStr=boolean
  AND11 : Logic  Operator=OR  AllPortsSameDT=off  OutDataTypeStr=boolean
  Bitwise AND{,1..4} (5 alike) : simulink/Logic and Bit Operations/Bitwise Operator  logicop=AND  UseBitMask=on  BitMask=bin2dec('11111111')  BitMaskRealWorld=Stored Integer
  Bitwise AND10 : simulink/Logic and Bit Operations/Bitwise Operator  logicop=AND  UseBitMask=on  BitMask=bin2dec('00100000')  BitMaskRealWorld=Stored Integer
  Bitwise AND5 : simulink/Logic and Bit Operations/Bitwise Operator  logicop=AND  UseBitMask=on  BitMask=bin2dec('00000001')  BitMaskRealWorld=Stored Integer
  Bitwise AND6 : simulink/Logic and Bit Operations/Bitwise Operator  logicop=AND  UseBitMask=on  BitMask=bin2dec('00000010')  BitMaskRealWorld=Stored Integer
  Bitwise AND7 : simulink/Logic and Bit Operations/Bitwise Operator  logicop=AND  UseBitMask=on  BitMask=bin2dec('00000100')  BitMaskRealWorld=Stored Integer
  Bitwise AND8 : simulink/Logic and Bit Operations/Bitwise Operator  logicop=AND  UseBitMask=on  BitMask=bin2dec('00001000')  BitMaskRealWorld=Stored Integer
  Bitwise AND9 : simulink/Logic and Bit Operations/Bitwise Operator  logicop=AND  UseBitMask=on  BitMask=bin2dec('00010000')  BitMaskRealWorld=Stored Integer
  Bitwise OR2 : simulink/Logic and Bit Operations/Bitwise Operator  logicop=OR  UseBitMask=off  NumInputPorts=6  BitMask=bin2dec('00000000000000000000')  BitMaskRealWorld=Stored Integer
  Compare To Constant5 : simulink/Logic and Bit Operations/Compare To Constant  relop===  const=0  OutDataTypeStr=boolean
  Constant : Constant  OutDataTypeStr=uint8
  Constant1 : Constant  Value=2  OutDataTypeStr=uint8
  Constant2 : Constant  Value=3  OutDataTypeStr=uint8
  Constant3 : Constant  Value=4  OutDataTypeStr=uint8
  Constant4 : Constant  Value=5  OutDataTypeStr=uint8
  Constant5 : Constant  Value=7  OutDataTypeStr=uint8
  Data Type Conversion{,1..5} (6 alike) : DataTypeConversion  OutDataTypeStr=uint8
  Data Type Conversion{6..11} (6 alike) : DataTypeConversion  OutDataTypeStr=boolean
  Detect Change1 : simulink/Logic and Bit Operations/Detect Change  vinit=0  OutDataTypeStr=boolean
  Detect Increase : simulink/Logic and Bit Operations/Detect Increase  vinit=0.0  OutDataTypeStr=boolean
  Multiport Switch : MultiPortSwitch  Inputs=7  DataPortForDefault=Additional data port  DiagnosticForDefault=None
  NOT : Logic  Operator=NOT  IconShape=distinctive  AllPortsSameDT=off  OutDataTypeStr=boolean
  NOT1 : Logic  Operator=NOT  IconShape=distinctive  AllPortsSameDT=off  OutDataTypeStr=boolean
  Relational Operator{,1..5} (6 alike) : RelationalOperator  Operator===  OutDataTypeStr=boolean  RndMeth=Simplest
  Shift Arithmetic1 : ArithShift  BitShiftNumber=4  BitShiftDirection=Left
  Shift Arithmetic10 : ArithShift  BitShiftNumber=5  BitShiftDirection=Right
  Shift Arithmetic2 : ArithShift  BitShiftNumber=5  BitShiftDirection=Left
  Shift Arithmetic3 : ArithShift  BitShiftNumber=1  BitShiftDirection=Right
  Shift Arithmetic4 : ArithShift  BitShiftNumber=2  BitShiftDirection=Right
  Shift Arithmetic5 : ArithShift  BitShiftNumber=3  BitShiftDirection=Right
  Shift Arithmetic6 : ArithShift  BitShiftNumber=1  BitShiftDirection=Left
  Shift Arithmetic7 : ArithShift  BitShiftNumber=2  BitShiftDirection=Left
  Shift Arithmetic8 : ArithShift  BitShiftNumber=3  BitShiftDirection=Left
  Shift Arithmetic9 : ArithShift  BitShiftNumber=4  BitShiftDirection=Right
  Switch{,1..3,5,7,12..13} (8 alike) : Switch  Criteria=u2 ~= 0
  Switch{4,6,8..11} (6 alike) : Switch  Criteria=u2 > Threshold
  Unit Delay{1..4,6..14} (13 alike) : UnitDelay  SampleTime=-1  HasFrameUpgradeWarning=on
  Setting : Outport
  Set : Outport  Port=2
  wires:
  Default/1 -> Multiport Switch/7, Multiport Switch/9
  [Set7] -> Multiport Switch/8
  [Set5] -> Multiport Switch/6
  [Set4] -> Multiport Switch/5
  [Set3] -> Multiport Switch/4
  [Set2] -> Multiport Switch/3
  [Set1] -> Multiport Switch/2
  NOT1/1 -> Switch1/2
  Switch13/1 -> Switch10/1
  Multiport Switch/1 -> Switch1/3
  Loadbar/1 -> [Loadbar], Compare To Constant5/1
  Switch1/1 -> Switch/3
  UserNow/1 -> Multiport Switch/1, [UserNow], Detect Change1/1
  NOT/1 -> Switch/1
  iviCMD/1 -> Detect Increase/1
  [Set] -> Switch13/1
  [Loadbar] -> Switch4/2
  [Set] -> Switch12/1
  [UserNow] -> Relational Operator5/1
  Constant5/1 -> Relational Operator5/2
  [UserNow] -> Relational Operator/1
  [UserNow] -> Relational Operator1/1
  [Loadbar] -> Switch10/2
  Constant2/1 -> Relational Operator2/2
  [Loadbar] -> Switch11/2
  [Set] -> Switch3/1
  Constant/1 -> Relational Operator/2
  [Loadbar] -> Switch9/2
  [UserNow] -> Relational Operator2/1
  [UserNow] -> Relational Operator3/1
  Constant3/1 -> Relational Operator3/2
  [Set] -> Switch2/1
  [UserNow] -> Relational Operator4/1
  Constant1/1 -> Relational Operator1/2
  [Set] -> Switch7/1
  [Loadbar] -> Switch6/2
  [Set] -> Switch5/1
  [Loadbar] -> Switch8/2
  Constant4/1 -> Relational Operator4/2
  Compare To Constant5/1 -> AND11/1
  AND11/1 -> NOT1/1
  Switch/1 -> Unit Delay7/1
  Switch8/1 -> [Set1], Unit Delay6/1
  Switch2/1 -> Switch8/1
  Switch3/1 -> Switch4/1
  Switch4/1 -> [Set2], Unit Delay1/1
  Switch6/1 -> [Set3], Unit Delay11/1
  Switch5/1 -> Switch6/1
  Switch7/1 -> Switch9/1
  Switch9/1 -> [Set4], Unit Delay12/1
  Switch10/1 -> [Set5], Unit Delay13/1
  Switch12/1 -> Switch11/1
  Switch11/1 -> [Set7], Unit Delay14/1
  Unit Delay7/1 -> Setting/1, NOT/1, [Set], Switch1/1
  Relational Operator2/1 -> Unit Delay10/1
  Relational Operator3/1 -> Unit Delay2/1
  Relational Operator4/1 -> Unit Delay3/1
  Relational Operator5/1 -> Unit Delay4/1
  Data Type Conversion2/1 -> Shift Arithmetic7/1
  Data Type Conversion5/1 -> Shift Arithmetic2/1
  [Set4] -> Data Type Conversion3/1
  Shift Arithmetic8/1 -> Bitwise AND/1
  Shift Arithmetic2/1 -> Bitwise AND4/1
  Bitwise AND3/1 -> Bitwise OR2/5
  Bitwise AND1/1 -> Bitwise OR2/3
  Bitwise AND2/1 -> Bitwise OR2/2
  Shift Arithmetic6/1 -> Bitwise AND2/1
  Data Type Conversion4/1 -> Shift Arithmetic1/1
  Shift Arithmetic7/1 -> Bitwise AND1/1
  Shift Arithmetic1/1 -> Bitwise AND3/1
  [Set7] -> Data Type Conversion5/1
  Data Type Conversion/1 -> Bitwise OR2/1
  [Set2] -> Data Type Conversion1/1
  Data Type Conversion3/1 -> Shift Arithmetic8/1
  [Set1] -> Data Type Conversion/1
  [Set5] -> Data Type Conversion4/1
  Bitwise AND/1 -> Bitwise OR2/4
  Data Type Conversion1/1 -> Shift Arithmetic6/1
  Bitwise AND4/1 -> Bitwise OR2/6
  [Set3] -> Data Type Conversion2/1
  Bitwise OR2/1 -> Set/1
  Bitwise AND8/1 -> Shift Arithmetic5/1
  Bitwise AND6/1 -> Shift Arithmetic3/1
  Bitwise AND9/1 -> Shift Arithmetic9/1
  Bitwise AND10/1 -> Shift Arithmetic10/1
  Shift Arithmetic4/1 -> Data Type Conversion8/1
  Shift Arithmetic10/1 -> Data Type Conversion11/1
  Bitwise AND5/1 -> Data Type Conversion6/1
  Shift Arithmetic3/1 -> Data Type Conversion7/1
  Bitwise AND7/1 -> Shift Arithmetic4/1
  Shift Arithmetic9/1 -> Data Type Conversion10/1
  Shift Arithmetic5/1 -> Data Type Conversion9/1
  EEP_Set/1 -> [EEP_Set]
  [EEP_Set] -> Bitwise AND5/1
  [EEP_Set] -> Bitwise AND6/1
  [EEP_Set] -> Bitwise AND7/1
  [EEP_Set] -> Bitwise AND8/1
  [EEP_Set] -> Bitwise AND9/1
  [EEP_Set] -> Bitwise AND10/1
  Data Type Conversion6/1 -> [EEP_Set1]
  Data Type Conversion7/1 -> [EEP_Set2]
  Data Type Conversion8/1 -> [EEP_Set3]
  Data Type Conversion9/1 -> [EEP_Set4]
  Data Type Conversion10/1 -> [EEP_Set5]
  Data Type Conversion11/1 -> [EEP_Set6]
  [EEP_Set1] -> Switch8/3
  [EEP_Set2] -> Switch4/3
  [EEP_Set3] -> Switch6/3
  [EEP_Set4] -> Switch9/3
  [EEP_Set5] -> Switch10/3
  [EEP_Set6] -> Switch11/3
  Relational Operator/1 -> Unit Delay8/1
  Relational Operator1/1 -> Unit Delay9/1
  Unit Delay6/1 -> Switch2/3
  Unit Delay1/1 -> Switch3/3
  Unit Delay8/1 -> Switch2/2
  Unit Delay9/1 -> Switch3/2
  Unit Delay10/1 -> Switch5/2
  Unit Delay11/1 -> Switch5/3
  Unit Delay2/1 -> Switch7/2
  Unit Delay12/1 -> Switch7/3
  Unit Delay3/1 -> Switch13/2
  Unit Delay13/1 -> Switch13/3
  Unit Delay4/1 -> Switch12/2
  Unit Delay14/1 -> Switch12/3
  AND/1 -> Switch/2
  Detect Increase/1 -> AND/2
  [Loadbar] -> AND/1
  Detect Change1/1 -> AND11/2

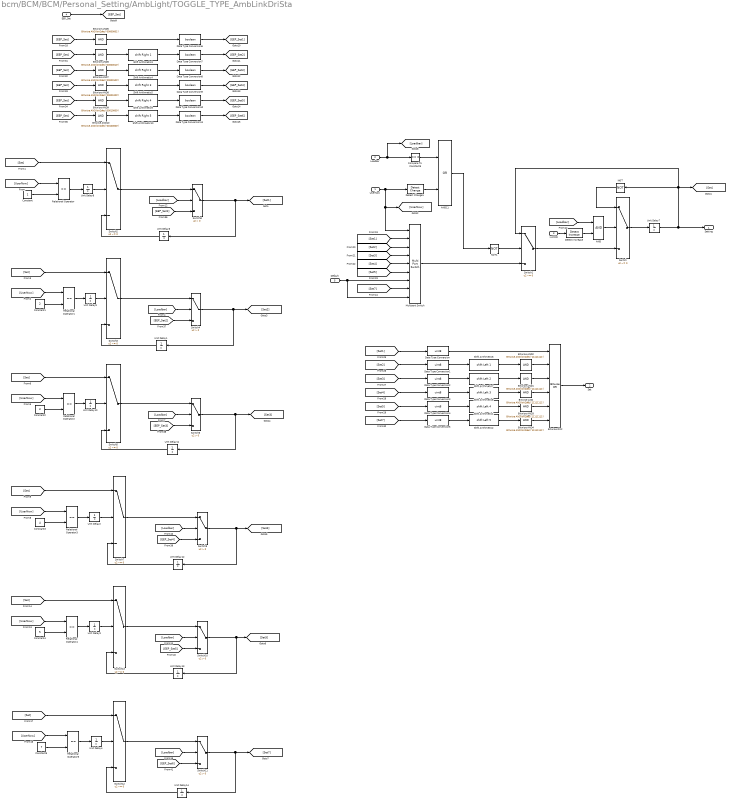
== system bcm/BCM/BCM/Personal_Setting/AmbLight/TOGGLE_TYPE_AmbLinkDriSta ==
  UserNow : Inport
  Loadbar : Inport  Port=2
  iviCMD : Inport  Port=3
  EEP_Set : Inport  Port=4
  Default : Inport  Port=5
  AND : Logic  AllPortsSameDT=off  OutDataTypeStr=boolean
  AND11 : Logic  Operator=OR  AllPortsSameDT=off  OutDataTypeStr=boolean
  Bitwise AND{,1..4} (5 alike) : simulink/Logic and Bit Operations/Bitwise Operator  logicop=AND  UseBitMask=on  BitMask=bin2dec('11111111')  BitMaskRealWorld=Stored Integer
  Bitwise AND10 : simulink/Logic and Bit Operations/Bitwise Operator  logicop=AND  UseBitMask=on  BitMask=bin2dec('00100000')  BitMaskRealWorld=Stored Integer
  Bitwise AND5 : simulink/Logic and Bit Operations/Bitwise Operator  logicop=AND  UseBitMask=on  BitMask=bin2dec('00000001')  BitMaskRealWorld=Stored Integer
  Bitwise AND6 : simulink/Logic and Bit Operations/Bitwise Operator  logicop=AND  UseBitMask=on  BitMask=bin2dec('00000010')  BitMaskRealWorld=Stored Integer
  Bitwise AND7 : simulink/Logic and Bit Operations/Bitwise Operator  logicop=AND  UseBitMask=on  BitMask=bin2dec('00000100')  BitMaskRealWorld=Stored Integer
  Bitwise AND8 : simulink/Logic and Bit Operations/Bitwise Operator  logicop=AND  UseBitMask=on  BitMask=bin2dec('00001000')  BitMaskRealWorld=Stored Integer
  Bitwise AND9 : simulink/Logic and Bit Operations/Bitwise Operator  logicop=AND  UseBitMask=on  BitMask=bin2dec('00010000')  BitMaskRealWorld=Stored Integer
  Bitwise OR2 : simulink/Logic and Bit Operations/Bitwise Operator  logicop=OR  UseBitMask=off  NumInputPorts=6  BitMask=bin2dec('00000000000000000000')  BitMaskRealWorld=Stored Integer
  Compare To Constant5 : simulink/Logic and Bit Operations/Compare To Constant  relop===  const=0  OutDataTypeStr=boolean
  Constant : Constant  OutDataTypeStr=uint8
  Constant1 : Constant  Value=2  OutDataTypeStr=uint8
  Constant2 : Constant  Value=3  OutDataTypeStr=uint8
  Constant3 : Constant  Value=4  OutDataTypeStr=uint8
  Constant4 : Constant  Value=5  OutDataTypeStr=uint8
  Constant5 : Constant  Value=7  OutDataTypeStr=uint8
  Data Type Conversion{,1..5} (6 alike) : DataTypeConversion  OutDataTypeStr=uint8
  Data Type Conversion{6..11} (6 alike) : DataTypeConversion  OutDataTypeStr=boolean
  Detect Change1 : simulink/Logic and Bit Operations/Detect Change  vinit=0  OutDataTypeStr=boolean
  Detect Increase : simulink/Logic and Bit Operations/Detect Increase  vinit=0.0  OutDataTypeStr=boolean
  Multiport Switch : MultiPortSwitch  Inputs=7  DataPortForDefault=Additional data port  DiagnosticForDefault=None
  NOT : Logic  Operator=NOT  IconShape=distinctive  AllPortsSameDT=off  OutDataTypeStr=boolean
  NOT1 : Logic  Operator=NOT  IconShape=distinctive  AllPortsSameDT=off  OutDataTypeStr=boolean
  Relational Operator{,1..5} (6 alike) : RelationalOperator  Operator===  OutDataTypeStr=boolean  RndMeth=Simplest
  Shift Arithmetic1 : ArithShift  BitShiftNumber=4  BitShiftDirection=Left
  Shift Arithmetic10 : ArithShift  BitShiftNumber=5  BitShiftDirection=Right
  Shift Arithmetic2 : ArithShift  BitShiftNumber=5  BitShiftDirection=Left
  Shift Arithmetic3 : ArithShift  BitShiftNumber=1  BitShiftDirection=Right
  Shift Arithmetic4 : ArithShift  BitShiftNumber=2  BitShiftDirection=Right
  Shift Arithmetic5 : ArithShift  BitShiftNumber=3  BitShiftDirection=Right
  Shift Arithmetic6 : ArithShift  BitShiftNumber=1  BitShiftDirection=Left
  Shift Arithmetic7 : ArithShift  BitShiftNumber=2  BitShiftDirection=Left
  Shift Arithmetic8 : ArithShift  BitShiftNumber=3  BitShiftDirection=Left
  Shift Arithmetic9 : ArithShift  BitShiftNumber=4  BitShiftDirection=Right
  Switch{,1..3,5,7,12..13} (8 alike) : Switch  Criteria=u2 ~= 0
  Switch{4,6,8..11} (6 alike) : Switch  Criteria=u2 > Threshold
  Unit Delay{1..4,6..14} (13 alike) : UnitDelay  SampleTime=-1  HasFrameUpgradeWarning=on
  Setting : Outport
  Set : Outport  Port=2
  wires:
  Default/1 -> Multiport Switch/7, Multiport Switch/9
  [Set7] -> Multiport Switch/8
  [Set5] -> Multiport Switch/6
  [Set4] -> Multiport Switch/5
  [Set3] -> Multiport Switch/4
  [Set2] -> Multiport Switch/3
  [Set1] -> Multiport Switch/2
  NOT1/1 -> Switch1/2
  Switch13/1 -> Switch10/1
  Detect Change1/1 -> AND11/2
  Multiport Switch/1 -> Switch1/3
  Loadbar/1 -> [Loadbar], Compare To Constant5/1
  Switch1/1 -> Switch/3
  UserNow/1 -> Multiport Switch/1, [UserNow], Detect Change1/1
  NOT/1 -> Switch/1
  iviCMD/1 -> Detect Increase/1
  [Set] -> Switch13/1
  [Loadbar] -> Switch4/2
  [Set] -> Switch12/1
  [UserNow] -> Relational Operator5/1
  Constant5/1 -> Relational Operator5/2
  [UserNow] -> Relational Operator/1
  [UserNow] -> Relational Operator1/1
  [Loadbar] -> Switch10/2
  Constant2/1 -> Relational Operator2/2
  [Loadbar] -> Switch11/2
  [Set] -> Switch3/1
  Constant/1 -> Relational Operator/2
  [Loadbar] -> Switch9/2
  [UserNow] -> Relational Operator2/1
  [UserNow] -> Relational Operator3/1
  Constant3/1 -> Relational Operator3/2
  [Set] -> Switch2/1
  [UserNow] -> Relational Operator4/1
  Constant1/1 -> Relational Operator1/2
  [Set] -> Switch7/1
  [Loadbar] -> Switch6/2
  [Set] -> Switch5/1
  [Loadbar] -> Switch8/2
  Constant4/1 -> Relational Operator4/2
  Compare To Constant5/1 -> AND11/1
  AND11/1 -> NOT1/1
  Switch/1 -> Unit Delay7/1
  Switch8/1 -> [Set1], Unit Delay6/1
  Switch2/1 -> Switch8/1
  Switch3/1 -> Switch4/1
  Switch4/1 -> [Set2], Unit Delay1/1
  Switch6/1 -> [Set3], Unit Delay11/1
  Switch5/1 -> Switch6/1
  Switch7/1 -> Switch9/1
  Switch9/1 -> [Set4], Unit Delay12/1
  Switch10/1 -> [Set5], Unit Delay13/1
  Switch12/1 -> Switch11/1
  Switch11/1 -> [Set7], Unit Delay14/1
  Unit Delay7/1 -> Setting/1, NOT/1, [Set], Switch1/1
  Relational Operator2/1 -> Unit Delay10/1
  Relational Operator3/1 -> Unit Delay2/1
  Relational Operator4/1 -> Unit Delay3/1
  Relational Operator5/1 -> Unit Delay4/1
  Data Type Conversion2/1 -> Shift Arithmetic7/1
  Data Type Conversion5/1 -> Shift Arithmetic2/1
  [Set4] -> Data Type Conversion3/1
  Shift Arithmetic8/1 -> Bitwise AND/1
  Shift Arithmetic2/1 -> Bitwise AND4/1
  Bitwise AND3/1 -> Bitwise OR2/5
  Bitwise AND1/1 -> Bitwise OR2/3
  Bitwise AND2/1 -> Bitwise OR2/2
  Shift Arithmetic6/1 -> Bitwise AND2/1
  Data Type Conversion4/1 -> Shift Arithmetic1/1
  Shift Arithmetic7/1 -> Bitwise AND1/1
  Shift Arithmetic1/1 -> Bitwise AND3/1
  [Set7] -> Data Type Conversion5/1
  Data Type Conversion/1 -> Bitwise OR2/1
  [Set2] -> Data Type Conversion1/1
  Data Type Conversion3/1 -> Shift Arithmetic8/1
  [Set1] -> Data Type Conversion/1
  [Set5] -> Data Type Conversion4/1
  Bitwise AND/1 -> Bitwise OR2/4
  Data Type Conversion1/1 -> Shift Arithmetic6/1
  Bitwise AND4/1 -> Bitwise OR2/6
  [Set3] -> Data Type Conversion2/1
  Bitwise OR2/1 -> Set/1
  Bitwise AND8/1 -> Shift Arithmetic5/1
  Bitwise AND6/1 -> Shift Arithmetic3/1
  Bitwise AND9/1 -> Shift Arithmetic9/1
  Bitwise AND10/1 -> Shift Arithmetic10/1
  Shift Arithmetic4/1 -> Data Type Conversion8/1
  Shift Arithmetic10/1 -> Data Type Conversion11/1
  Bitwise AND5/1 -> Data Type Conversion6/1
  Shift Arithmetic3/1 -> Data Type Conversion7/1
  Bitwise AND7/1 -> Shift Arithmetic4/1
  Shift Arithmetic9/1 -> Data Type Conversion10/1
  Shift Arithmetic5/1 -> Data Type Conversion9/1
  EEP_Set/1 -> [EEP_Set]
  [EEP_Set] -> Bitwise AND5/1
  [EEP_Set] -> Bitwise AND6/1
  [EEP_Set] -> Bitwise AND7/1
  [EEP_Set] -> Bitwise AND8/1
  [EEP_Set] -> Bitwise AND9/1
  [EEP_Set] -> Bitwise AND10/1
  Data Type Conversion6/1 -> [EEP_Set1]
  Data Type Conversion7/1 -> [EEP_Set2]
  Data Type Conversion8/1 -> [EEP_Set3]
  Data Type Conversion9/1 -> [EEP_Set4]
  Data Type Conversion10/1 -> [EEP_Set5]
  Data Type Conversion11/1 -> [EEP_Set6]
  [EEP_Set1] -> Switch8/3
  [EEP_Set2] -> Switch4/3
  [EEP_Set3] -> Switch6/3
  [EEP_Set4] -> Switch9/3
  [EEP_Set5] -> Switch10/3
  [EEP_Set6] -> Switch11/3
  Relational Operator/1 -> Unit Delay8/1
  Relational Operator1/1 -> Unit Delay9/1
  Unit Delay6/1 -> Switch2/3
  Unit Delay1/1 -> Switch3/3
  Unit Delay8/1 -> Switch2/2
  Unit Delay9/1 -> Switch3/2
  Unit Delay10/1 -> Switch5/2
  Unit Delay11/1 -> Switch5/3
  Unit Delay2/1 -> Switch7/2
  Unit Delay12/1 -> Switch7/3
  Unit Delay3/1 -> Switch13/2
  Unit Delay13/1 -> Switch13/3
  Unit Delay4/1 -> Switch12/2
  Unit Delay14/1 -> Switch12/3
  AND/1 -> Switch/2
  Detect Increase/1 -> AND/2
  [Loadbar] -> AND/1
